simulink model "gm_uz_ninephase_VSD_transformation"  (R2021b)
settings: Solver=FixedStepAuto  StartTime=0.0  StopTime=inf  RelTol=1e-3
undefined symbols (not defined in the file or in its folder): a, b, c
libraries: hdlsllib x90, simulink x32, hdlmdlgenlib x20, dspsigops x7
(part 1 of 6)
settings Model: Creator=ts  LastModifiedBy=valen
settings SolverCC: AlgebraicLoopSolver=TrustRegion  AutoInsertRateTranBlk=on
settings DataIOCC: LimitDataPoints=on  SaveOutput=off  SaveTime=off
settings OptimizationCC: BlockReduction=off  ConditionallyExecuteInputs=off  DefaultParameterBehavior=Inlined  InheritOutputTypeSmallerThanSingle=on  LifeSpan=inf
settings DebuggingCC: AlgebraicLoopMsg=error  ArtificialAlgebraicLoopMsg=none  InheritedTsInSrcMsg=none  SingleTaskRateTransMsg=error  AllowSymbolicDim=off  StrictBusMsg=ErrorOnBusTreatedAsVector  SFUnexpectedBacktrackingDiag=warning  SFNoUnconditionalDefaultTransitionDiag=warning  SFExecutionAtInitializationDiag=none  SFMachineParentedDataDiag=warning  ArithmeticOperatorsInVariantConditions=warning
settings HardwareCC: ProdBitPerPointer=32  ProdBitPerSizeT=32  ProdBitPerPtrDiffT=32  ProdLargestAtomicFloat=None  ProdIntDivRoundTo=Undefined  ProdEndianess=Unspecified  ProdWordSize=32  ProdHWDeviceType=ASIC/FPGA->ASIC/FPGA  ProdEqTarget=off
settings SFSimCC: SimUseLocalCustomCode=off  CustomCodeUndefinedFunction=UseInterfaceOnly
settings RTWCC: RTWUseLocalCustomCode=off
settings CodeAppCC: StateflowObjectComments=on
settings GRTTargetCC: TargetLangStandard=C89/C90 (ANSI)
settings ConfigComp: CovScope=ReferencedModels  CovMetricSettings=dw  CovSaveCumulativeToWorkspaceVar=on  CovSaveSingleToWorkspaceVar=on  CovExternalEMLEnable=off  CovSFcnEnable=off

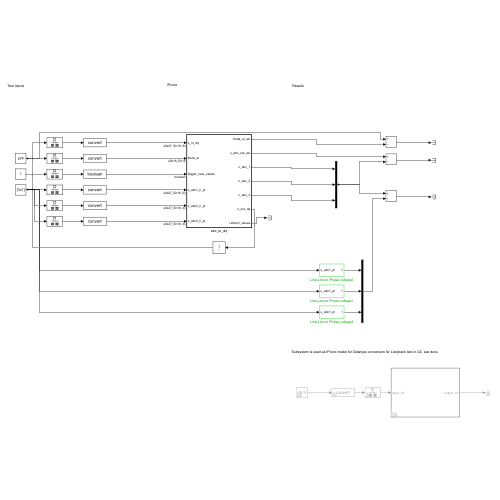
[thumbnail: Simulink's stored preview of the top-level diagram]
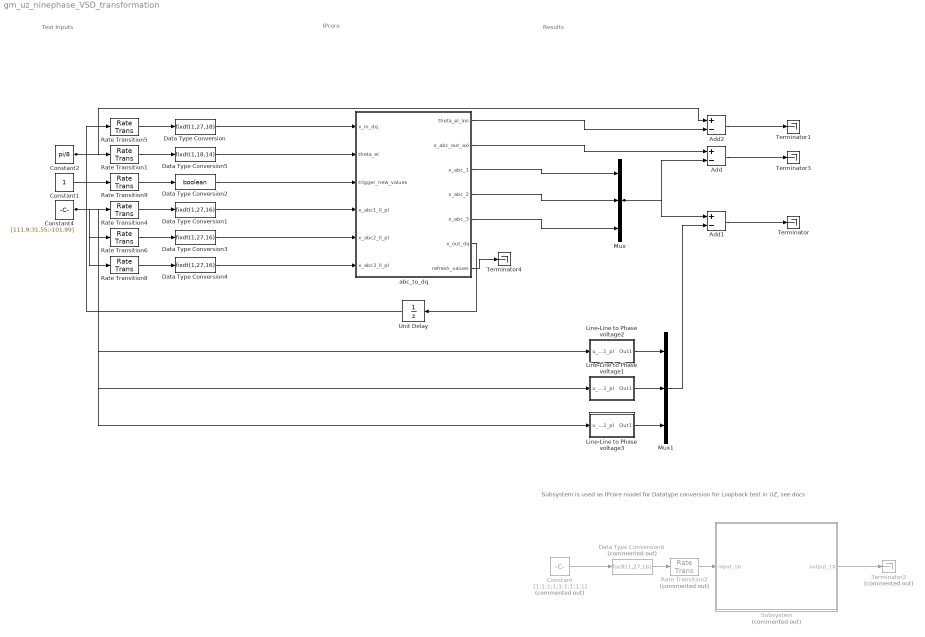
== system gm_uz_ninephase_VSD_transformation ==
  note: IPcore
  note: Test Inputs
  note: Results
  note: Subsystem is used as IPcore model for Datatype conversion for Loopback test in UZ, see docs
  Add : Sum  Inputs=+-
  Add1 : Sum  Inputs=+-
  Add2 : Sum  Inputs=+-
  Constant : Constant  Commented=on  Value=[1;1;1;1;1;1;1;1;1]
  Constant1 : Constant
  Constant2 : Constant  Value=pi/8
  Constant4 : Constant  Value=[111.9;31.55;-101.99]
  Data Type Conversion : DataTypeConversion  OutDataTypeStr=fixdt(1,27,18)
  Data Type Conversion1 : DataTypeConversion  OutDataTypeStr=fixdt(1,27,16)
  Data Type Conversion2 : DataTypeConversion  OutDataTypeStr=boolean
  Data Type Conversion3 : DataTypeConversion  OutDataTypeStr=fixdt(1,27,16)
  Data Type Conversion4 : DataTypeConversion  OutDataTypeStr=fixdt(1,27,16)
  Data Type Conversion5 : DataTypeConversion  OutDataTypeStr=fixdt(1,18,14)
  Data Type Conversion6 : DataTypeConversion  Commented=on  OutDataTypeStr=fixdt(1,27,16)
  Line-Line to Phase voltage1 : Subsystem
  Line-Line to Phase voltage2 : Subsystem
  Line-Line to Phase voltage3 : Subsystem
  Mux : Mux  Inputs=3
  Mux1 : Mux  Inputs=3
  Rate Transition{1,4..6,8..9} (6 alike) : RateTransition  OutPortSampleTime=ts_uz_ninephase_VSD_transformation
  Rate Transition2 : RateTransition  Commented=on  OutPortSampleTime=ts_uz_ninephase_VSD_transformation
  Subsystem : Subsystem  Commented=on  TreatAsAtomicUnit=on
  Terminator{,1,3..4} (4 alike) : Terminator
  Terminator2 : Terminator  Commented=on
  Unit Delay : UnitDelay  SampleTime=-1  HasFrameUpgradeWarning=on
  abc_to_dq : Subsystem  TreatAsAtomicUnit=on
  wires:
  abc_to_dq/7(refresh_values) -> Terminator4/1
  Rate Transition2/1 -> Subsystem/1(input_16)
  Data Type Conversion6/1 -> Rate Transition2/1
  Constant/1 -> Data Type Conversion6/1
  Subsystem/1(output_18) -> Terminator2/1
  Line-Line to Phase voltage3/1(Out1) -> Mux1/3
  Line-Line to Phase voltage1/1(Out1) -> Mux1/2
  Line-Line to Phase voltage2/1(Out1) -> Mux1/1
  Unit Delay/1 -> Rate Transition5/1
  Add/1 -> Terminator3/1
  Constant4/1 -> Rate Transition4/1, Rate Transition6/1, Line-Line to Phase voltage1/1(u_abc1_pl), Line-Line to Phase voltage3/1(u_abc1_pl), Line-Line to Phase voltage2/1(u_abc1_pl), Rate Transition8/1
  Add2/1 -> Terminator1/1
  abc_to_dq/1(theta_el_axi) -> Add2/2
  Add1/1 -> Terminator/1
  Mux1/1 -> Add1/2
  abc_to_dq/2(x_abc_out_axi) -> Add/1
  Mux/1 -> Add/2, Add1/1
  abc_to_dq/4(x_abc_2) -> Mux/2
  abc_to_dq/5(x_abc_3) -> Mux/3
  abc_to_dq/3(x_abc_1) -> Mux/1
  Constant2/1 -> Rate Transition1/1, Add2/1
  abc_to_dq/6(x_out_dq) -> Unit Delay/1
  Rate Transition1/1 -> Data Type Conversion5/1
  Data Type Conversion5/1 -> abc_to_dq/2(theta_el)
  Constant1/1 -> Rate Transition9/1
  Rate Transition9/1 -> Data Type Conversion2/1
  Data Type Conversion2/1 -> abc_to_dq/3(trigger_new_values)
  Rate Transition8/1 -> Data Type Conversion4/1
  Rate Transition6/1 -> Data Type Conversion3/1
  Rate Transition4/1 -> Data Type Conversion1/1
  Data Type Conversion3/1 -> abc_to_dq/5(x_abc2_ll_pl)
  Data Type Conversion4/1 -> abc_to_dq/6(x_abc3_ll_pl)
  Rate Transition5/1 -> Data Type Conversion/1
  Data Type Conversion1/1 -> abc_to_dq/4(x_abc1_ll_pl)
  Data Type Conversion/1 -> abc_to_dq/1(x_in_dq)

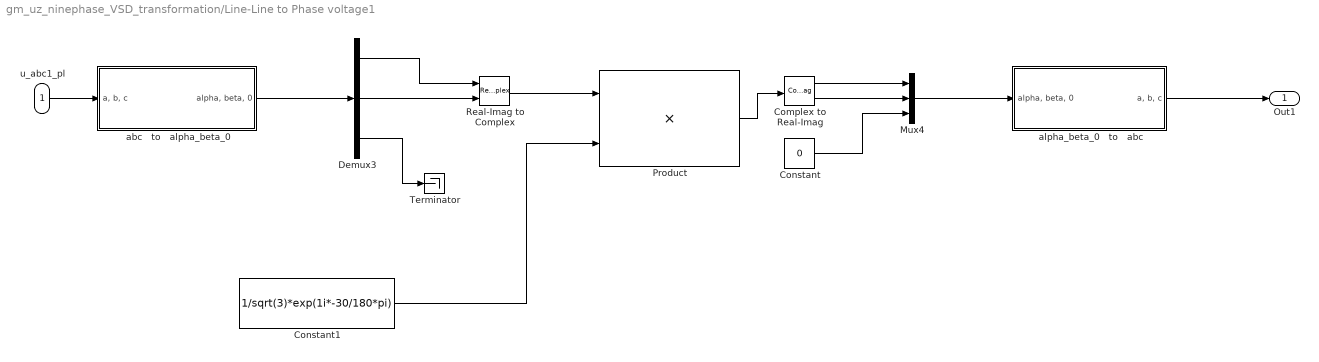
== system gm_uz_ninephase_VSD_transformation/Line-Line to Phase voltage1 ==
  u_abc1_pl : Inport
  Complex to Real-Imag : ComplexToRealImag
  Constant : Constant  Value=0  OutDataTypeStr=fixdt(1,27,16)  SampleTime=-1
  Constant1 : Constant  Value=1/sqrt(3)*exp(1i*-30/180*pi)  OutDataTypeStr=fixdt(1,18,16)  SampleTime=-1
  Demux3 : Demux  Outputs=3
  Mux4 : Mux  Inputs=3
  Product : Product  OutDataTypeStr=fixdt(1,27,16)
  Real-Imag to Complex : RealImagToComplex
  Terminator : Terminator
  abc   to   alpha_beta_0 : Subsystem
  alpha_beta_0   to   abc : Subsystem
  Out1 : Outport
  wires:
  Demux3/2 -> Real-Imag to Complex/2
  Complex to Real-Imag/1 -> Mux4/1
  Mux4/1 -> alpha_beta_0   to   abc/1("alpha, beta, 0  ")
  Product/1 -> Complex to Real-Imag/1
  Real-Imag to Complex/1 -> Product/1
  Demux3/1 -> Real-Imag to Complex/1
  Complex to Real-Imag/2 -> Mux4/2
  Constant/1 -> Mux4/3
  u_abc1_pl/1 -> abc   to   alpha_beta_0/1("a, b, c")
  Demux3/3 -> Terminator/1
  abc   to   alpha_beta_0/1("alpha, beta, 0 ") -> Demux3/1
  alpha_beta_0   to   abc/1("a, b, c") -> Out1/1
  Constant1/1 -> Product/2

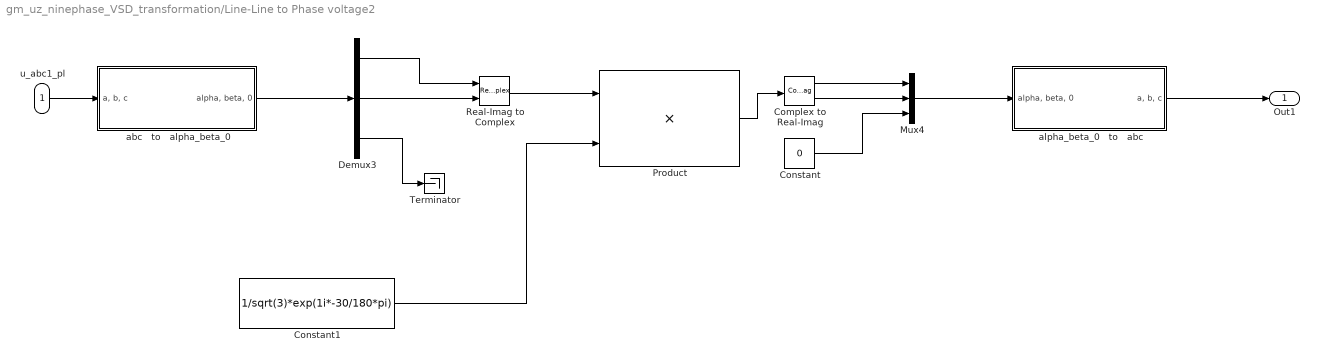
== system gm_uz_ninephase_VSD_transformation/Line-Line to Phase voltage2 ==
  u_abc1_pl : Inport
  Complex to Real-Imag : ComplexToRealImag
  Constant : Constant  Value=0  OutDataTypeStr=fixdt(1,27,16)  SampleTime=-1
  Constant1 : Constant  Value=1/sqrt(3)*exp(1i*-30/180*pi)  OutDataTypeStr=fixdt(1,18,16)  SampleTime=-1
  Demux3 : Demux  Outputs=3
  Mux4 : Mux  Inputs=3
  Product : Product  OutDataTypeStr=fixdt(1,27,16)
  Real-Imag to Complex : RealImagToComplex
  Terminator : Terminator
  abc   to   alpha_beta_0 : Subsystem
  alpha_beta_0   to   abc : Subsystem
  Out1 : Outport
  wires:
  Constant1/1 -> Product/2
  alpha_beta_0   to   abc/1("a, b, c") -> Out1/1
  abc   to   alpha_beta_0/1("alpha, beta, 0 ") -> Demux3/1
  Demux3/3 -> Terminator/1
  u_abc1_pl/1 -> abc   to   alpha_beta_0/1("a, b, c")
  Constant/1 -> Mux4/3
  Complex to Real-Imag/2 -> Mux4/2
  Demux3/1 -> Real-Imag to Complex/1
  Real-Imag to Complex/1 -> Product/1
  Product/1 -> Complex to Real-Imag/1
  Mux4/1 -> alpha_beta_0   to   abc/1("alpha, beta, 0  ")
  Complex to Real-Imag/1 -> Mux4/1
  Demux3/2 -> Real-Imag to Complex/2

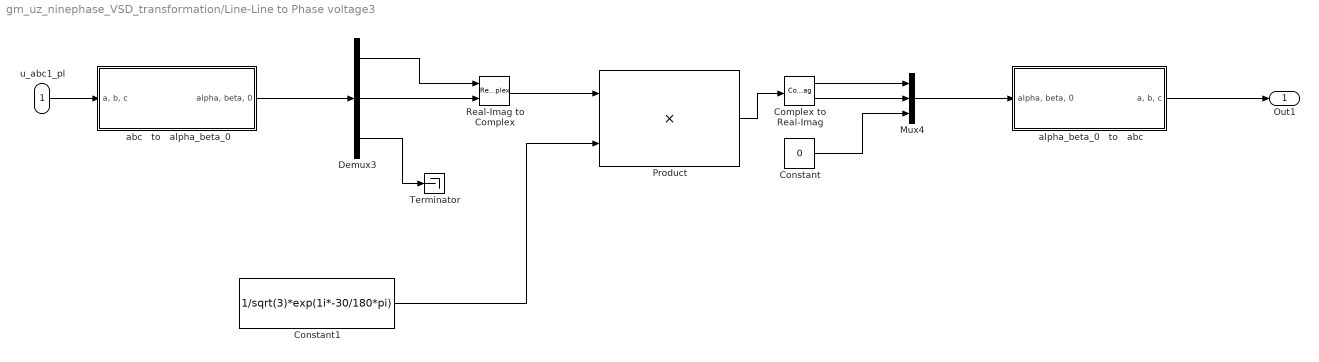
== system gm_uz_ninephase_VSD_transformation/Line-Line to Phase voltage3 ==
  u_abc1_pl : Inport
  Complex to Real-Imag : ComplexToRealImag
  Constant : Constant  Value=0  OutDataTypeStr=fixdt(1,27,16)  SampleTime=-1
  Constant1 : Constant  Value=1/sqrt(3)*exp(1i*-30/180*pi)  OutDataTypeStr=fixdt(1,18,16)  SampleTime=-1
  Demux3 : Demux  Outputs=3
  Mux4 : Mux  Inputs=3
  Product : Product  OutDataTypeStr=fixdt(1,27,16)
  Real-Imag to Complex : RealImagToComplex
  Terminator : Terminator
  abc   to   alpha_beta_0 : Subsystem
  alpha_beta_0   to   abc : Subsystem
  Out1 : Outport
  wires:
  Constant1/1 -> Product/2
  alpha_beta_0   to   abc/1("a, b, c") -> Out1/1
  abc   to   alpha_beta_0/1("alpha, beta, 0 ") -> Demux3/1
  Demux3/3 -> Terminator/1
  u_abc1_pl/1 -> abc   to   alpha_beta_0/1("a, b, c")
  Constant/1 -> Mux4/3
  Complex to Real-Imag/2 -> Mux4/2
  Demux3/1 -> Real-Imag to Complex/1
  Real-Imag to Complex/1 -> Product/1
  Product/1 -> Complex to Real-Imag/1
  Mux4/1 -> alpha_beta_0   to   abc/1("alpha, beta, 0  ")
  Complex to Real-Imag/1 -> Mux4/1
  Demux3/2 -> Real-Imag to Complex/2

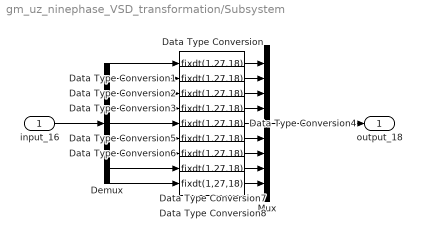
== system gm_uz_ninephase_VSD_transformation/Subsystem ==
  input_16 : Inport
  Data Type Conversion{,1..8} (9 alike) : DataTypeConversion  OutDataTypeStr=fixdt(1,27,18)
  Demux : Demux  Outputs=9
  Mux : Mux  Inputs=9
  output_18 : Outport
  wires:
  Mux/1 -> output_18/1
  Data Type Conversion8/1 -> Mux/9
  Data Type Conversion7/1 -> Mux/8
  Data Type Conversion6/1 -> Mux/7
  Data Type Conversion5/1 -> Mux/6
  Data Type Conversion4/1 -> Mux/5
  Data Type Conversion3/1 -> Mux/4
  Data Type Conversion2/1 -> Mux/3
  Data Type Conversion1/1 -> Mux/2
  Data Type Conversion/1 -> Mux/1
  Demux/9 -> Data Type Conversion8/1
  Demux/8 -> Data Type Conversion7/1
  Demux/7 -> Data Type Conversion6/1
  Demux/4 -> Data Type Conversion3/1
  Demux/5 -> Data Type Conversion4/1
  Demux/6 -> Data Type Conversion5/1
  Demux/3 -> Data Type Conversion2/1
  Demux/2 -> Data Type Conversion1/1
  Demux/1 -> Data Type Conversion/1
  input_16/1 -> Demux/1
